simulink model "Full_Adder"  (R2020a)
settings: Solver=VariableStepAuto  StartTime=0.0  StopTime=10.0  RelTol=1e-3
settings Model: Creator=ashwin  LastModifiedBy=ashwin

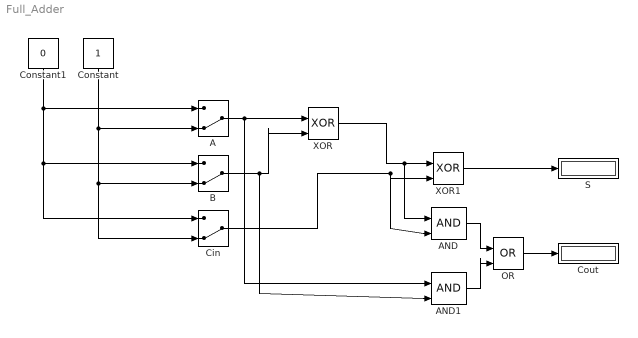
== system Full_Adder ==
  A : ManualSwitch  CurrentSetting=0
  AND : Logic  IconShape=distinctive  AllPortsSameDT=off  OutDataTypeStr=boolean
  AND1 : Logic  IconShape=distinctive  AllPortsSameDT=off  OutDataTypeStr=boolean
  B : ManualSwitch  CurrentSetting=0
  Cin : ManualSwitch  CurrentSetting=0
  Constant : Constant
  Constant1 : Constant  Value=0
  Cout : Display
  OR : Logic  Operator=OR  IconShape=distinctive  AllPortsSameDT=off  OutDataTypeStr=boolean
  S : Display
  XOR : Logic  Operator=XOR  IconShape=distinctive  AllPortsSameDT=off  OutDataTypeStr=boolean
  XOR1 : Logic  Operator=XOR  IconShape=distinctive  AllPortsSameDT=off  OutDataTypeStr=boolean
  wires:
  XOR/1 -> AND/1, XOR1/1
  A/1 -> AND1/1, XOR/1
  B/1 -> AND1/2, XOR/2
  Constant1/1 -> A/1, B/1, Cin/1
  Constant/1 -> A/2, Cin/2, B/2
  Cin/1 -> AND/2, XOR1/2
  XOR1/1 -> S/1
  AND1/1 -> OR/2
  AND/1 -> OR/1
  OR/1 -> Cout/1
